simulink model "ICE_Braking_System"  (R2017b)
settings: Solver=VariableStepAuto  StartTime=0.0  StopTime=1000.0  RelTol=1e-3
values from neighbouring files (symbols this model uses):
  g = 9.8    [ICE_Breaking_System_Variables.m]
  k = 10000    [ICE_Breaking_System_Variables.m]
  M1 = 10000    [ICE_Breaking_System_Variables.m]
  M2 = 15000    [ICE_Breaking_System_Variables.m]
  mu = 0.0015    [ICE_Breaking_System_Variables.m]
settings Model: Creator=vaibhav  LastModifiedBy=vaibhav

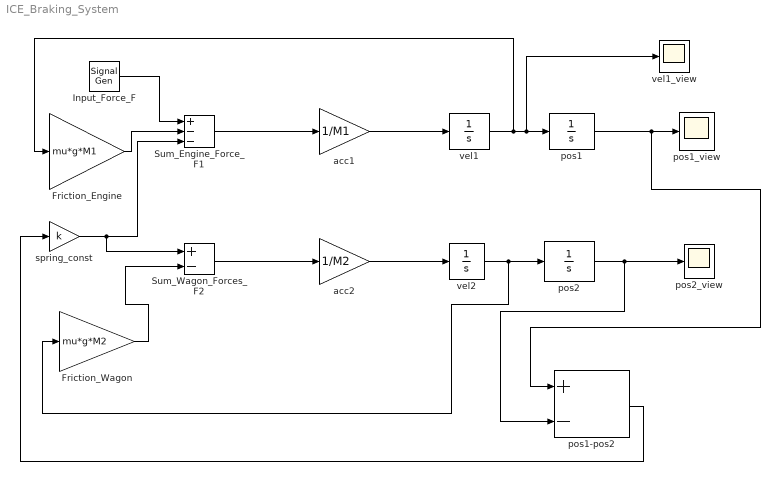
== system ICE_Braking_System ==
  Friction_Engine : Gain  Gain=mu*g*M1
  Friction_Wagon : Gain  Gain=mu*g*M2
  Input_Force_F : SignalGenerator  WaveForm=square  Amplitude=-1  Frequency=0.001
  Sum_Engine_Force_F1 : Sum  Inputs=+--
  Sum_Wagon_Forces_F2 : Sum  Inputs=+-
  acc1 : Gain  Gain=1/M1
  acc2 : Gain  Gain=1/M2
  pos1 : Integrator
  pos1-pos2 : Sum  Inputs=+-
  pos1_view : Scope
  pos2 : Integrator
  "pos2_view " : Scope
  spring_const : Gain  Gain=k
  vel1 : Integrator
  "vel1_view " : Scope
  vel2 : Integrator
  wires:
  Sum_Engine_Force_F1/1 -> acc1/1
  Sum_Wagon_Forces_F2/1 -> acc2/1
  acc1/1 -> vel1/1
  acc2/1 -> vel2/1
  vel1/1 -> Friction_Engine/1, "vel1_view "/1, pos1/1
  Input_Force_F/1 -> Sum_Engine_Force_F1/1
  pos1/1 -> pos1-pos2/1, pos1_view/1
  pos2/1 -> pos1-pos2/2, "pos2_view "/1
  pos1-pos2/1 -> spring_const/1
  spring_const/1 -> Sum_Wagon_Forces_F2/1, Sum_Engine_Force_F1/3
  Friction_Engine/1 -> Sum_Engine_Force_F1/2
  vel2/1 -> Friction_Wagon/1, pos2/1
  Friction_Wagon/1 -> Sum_Wagon_Forces_F2/2
